simulink model "pil_testing"  (R2016a)
settings: Solver=FixedStepAuto  StartTime=0.0  StopTime=inf  FixedStep=0.05  RelTol=1e-3
undefined symbols (not defined in the file): Serial_Port, Standard_Devices
libraries: sldrtlib x2
settings Model: SimulationMode=external  Creator=aless  LastModifiedBy=aless
settings SolverCC: EnableConcurrentExecution=on
settings DataIOCC: SaveFormat=StructureWithTime  SignalLogging=off  DSMLogging=off
settings OptimizationCC: BlockReduction=off  DefaultUnderspecifiedDataType=single  OptimizeBlockIOStorage=off  BufferReuse=off  GlobalBufferReuse=off  ExpressionFolding=off  LocalBlockOutputs=off
settings DebuggingCC: MultiTaskRateTransMsg=warning
settings HardwareCC: ProdBitPerLong=64  ProdLargestAtomicFloat=None  ProdHWDeviceType=Intel->x86-64  TargetBitPerLong=64  TargetBitPerPointer=64  TargetIntDivRoundTo=Zero  TargetEndianess=LittleEndian  TargetWordSize=64  TargetHWDeviceType=Intel->x86-64
settings RTWCC: SystemTargetFile=sldrt.tlc  TemplateMakefile=sldrt.tmf  Description=Simulink Desktop Real-Time  RTWVerbose=off  RTWCompilerOptimization=on
settings CodeAppCC: ForceParamTrailComments=on  MaxIdLength=95  OperatorAnnotations=on  MATLABSourceComments=on
settings SimulinkDesktopRealTimeCC: TargetPreCompLibLocation=C:\Program Files\MATLAB\R2016a\toolbox\sldrt\lib\win64  TargetLangStandard=C89/C90 (ANSI)  SupportVariableSizeSignals=off

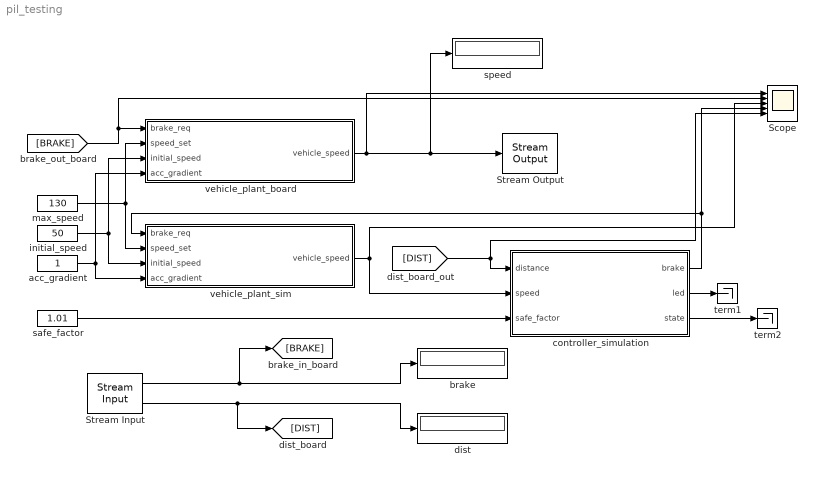
== system pil_testing ==
  Scope : Scope  NumInputPorts=5
  Stream Input : sldrtlib/Stream Input  SampleTime=0.1  MaxMissedTicks=10  ShowMissedTicks=off  YieldWhenWaiting=off  DrvName=Standard_Devices/Serial_Port  DrvAddress=5  DrvOptions=[9600 8 0 0 0 0 0 0]  DataTypes={'uint8','uint8'}  FormatString='%d %d'  Terminator='\n'  ShowReady=off  ShowError=off
      settings: AttributesFormatString=Standard Devices\nSerial Port [5h]
  Stream Output : sldrtlib/Stream Output  SampleTime=0.1  MaxMissedTicks=10  ShowMissedTicks=off  YieldWhenWaiting=off  DrvName=Standard_Devices/Serial_Port  DrvAddress=5  DrvOptions=[9600 8 0 0 0 0 0 0]  PortSizes=1  FormatString='%d\r'  ShowReady=off  ShowError=off  InitialValue=[]  FinalValue=[]
      settings: AttributesFormatString=Standard Devices\nSerial Port [5h]
  acc_gradient : Constant
  brake : Display
  controller_simulation : Subsystem
  dist : Display
  initial_speed : Constant  Value=50
  max_speed : Constant  Value=130
  safe_factor : Constant  Value=1.01
  speed : Display
  term1 : Terminator
  term2 : Terminator
  vehicle_plant_board : Subsystem
  vehicle_plant_sim : Subsystem
  wires:
  [BRAKE] -> vehicle_plant_board/1(brake_req), Scope/2
  safe_factor/1 -> controller_simulation/3(safe_factor)
  vehicle_plant_sim/1(vehicle_speed) -> controller_simulation/2(speed), Scope/3
  controller_simulation/2(led) -> term1/1
  controller_simulation/3(state) -> term2/1
  controller_simulation/1(brake) -> vehicle_plant_sim/1(brake_req), Scope/4
  vehicle_plant_board/1(vehicle_speed) -> speed/1, Stream Output/1, Scope/1
  max_speed/1 -> vehicle_plant_board/2(speed_set), vehicle_plant_sim/2(speed_set)
  initial_speed/1 -> vehicle_plant_board/3(initial_speed), vehicle_plant_sim/3(initial_speed)
  acc_gradient/1 -> vehicle_plant_board/4(acc_gradient), vehicle_plant_sim/4(acc_gradient)
  [DIST] -> controller_simulation/1(distance), Scope/5
  Stream Input/1 -> [BRAKE], brake/1
  Stream Input/2 -> dist/1, [DIST]

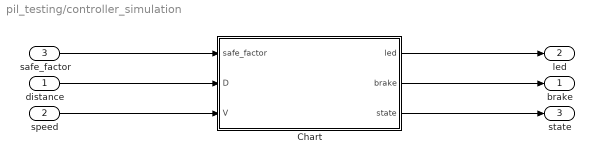
== system pil_testing/controller_simulation ==
  distance : Inport
  speed : Inport  Port=2
  safe_factor : Inport  Port=3
  Chart : Stateflow chart  TreatAsAtomicUnit=on
  brake : Outport
  led : Outport  Port=2
  state : Outport  Port=3
  wires:
  distance/1 -> Chart/2(D)
  speed/1 -> Chart/3(V)
  safe_factor/1 -> Chart/1(safe_factor)
  Chart/1(led) -> led/1
  Chart/2(brake) -> brake/1
  Chart/3(state) -> state/1

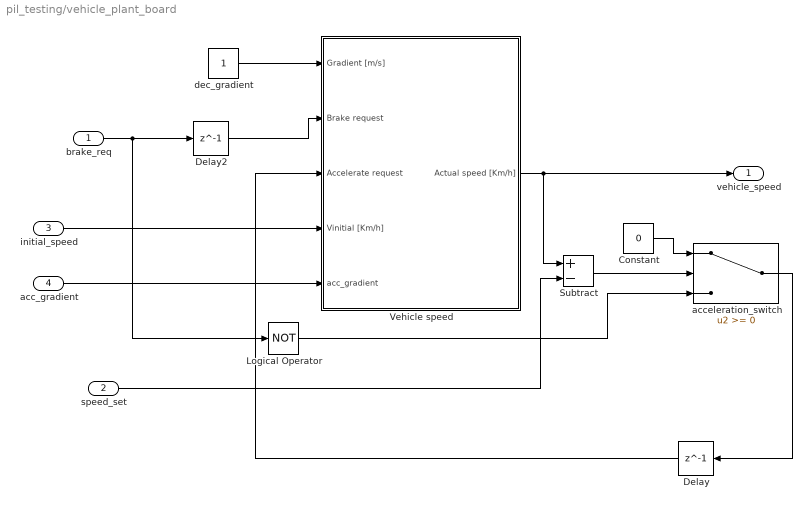
== system pil_testing/vehicle_plant_board ==
  brake_req : Inport
  speed_set : Inport  Port=2
  initial_speed : Inport  Port=3
  acc_gradient : Inport  Port=4
  Constant : Constant  Value=0
  Delay : Delay  DelayLength=1  InitialCondition=0
  Delay2 : Delay  DelayLength=1  InitialCondition=0
  Logical Operator : Logic  Operator=NOT  AllPortsSameDT=off  OutDataTypeStr=boolean
  Subtract : Sum  Inputs=+-
  Vehicle speed : Subsystem
  acceleration_switch : Switch  RndMeth=Nearest
  dec_gradient : Constant
  vehicle_speed : Outport
  wires:
  dec_gradient/1 -> Vehicle speed/1(Gradient [m/s])
  initial_speed/1 -> Vehicle speed/4(Vinitial [Km/h])
  Vehicle speed/1(Actual speed [Km/h]) -> vehicle_speed/1, Subtract/1
  Constant/1 -> acceleration_switch/1
  brake_req/1 -> Logical Operator/1, Delay2/1
  acceleration_switch/1 -> Delay/1
  Subtract/1 -> acceleration_switch/2
  speed_set/1 -> Subtract/2
  Delay2/1 -> Vehicle speed/2(Brake request)
  Logical Operator/1 -> acceleration_switch/3
  acc_gradient/1 -> Vehicle speed/5(acc_gradient)
  Delay/1 -> Vehicle speed/3(Accelerate request)

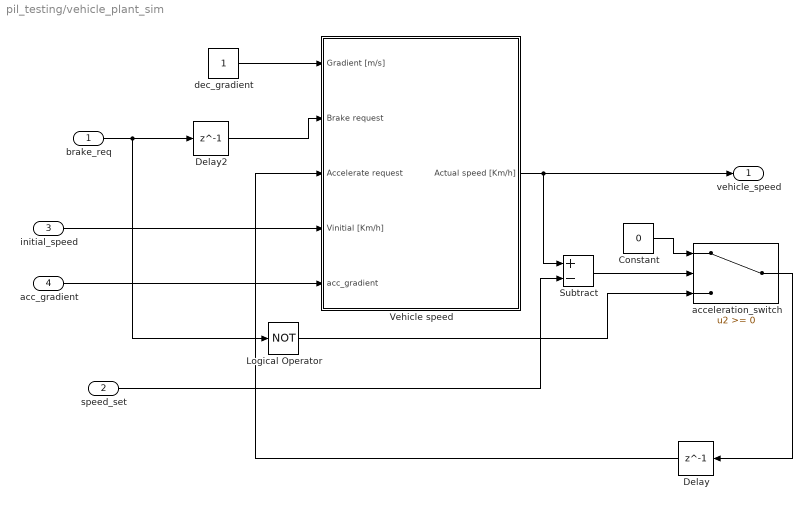
== system pil_testing/vehicle_plant_sim ==
  brake_req : Inport
  speed_set : Inport  Port=2
  initial_speed : Inport  Port=3
  acc_gradient : Inport  Port=4
  Constant : Constant  Value=0
  Delay : Delay  DelayLength=1  InitialCondition=0
  Delay2 : Delay  DelayLength=1  InitialCondition=0
  Logical Operator : Logic  Operator=NOT  AllPortsSameDT=off  OutDataTypeStr=boolean
  Subtract : Sum  Inputs=+-
  Vehicle speed : Subsystem
  acceleration_switch : Switch  RndMeth=Nearest
  dec_gradient : Constant
  vehicle_speed : Outport
  wires:
  dec_gradient/1 -> Vehicle speed/1(Gradient [m/s])
  initial_speed/1 -> Vehicle speed/4(Vinitial [Km/h])
  Vehicle speed/1(Actual speed [Km/h]) -> vehicle_speed/1, Subtract/1
  Constant/1 -> acceleration_switch/1
  brake_req/1 -> Logical Operator/1, Delay2/1
  acceleration_switch/1 -> Delay/1
  Subtract/1 -> acceleration_switch/2
  speed_set/1 -> Subtract/2
  Delay2/1 -> Vehicle speed/2(Brake request)
  Logical Operator/1 -> acceleration_switch/3
  acc_gradient/1 -> Vehicle speed/5(acc_gradient)
  Delay/1 -> Vehicle speed/3(Accelerate request)

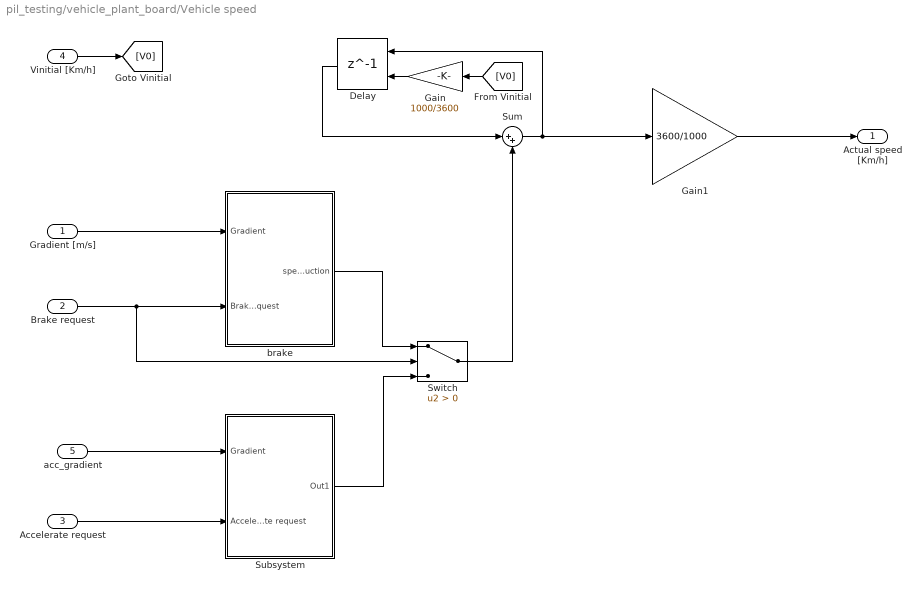
== system pil_testing/vehicle_plant_board/Vehicle speed ==
  Gradient [m/s] : Inport
  Brake request : Inport  Port=2
  Accelerate request : Inport  Port=3
  Vinitial [Km/h] : Inport  Port=4
  acc_gradient : Inport  Port=5
  Delay : Delay  DelayLength=1  InitialConditionSource=Input port  InitialCondition=0
      settings: InputPortMap=u0,p4
  Gain : Gain  Gain=1000/3600
  Gain1 : Gain  Gain=3600/1000
  Subsystem : Subsystem
  Sum : Sum  Inputs=|++
  Switch : Switch  Criteria=u2 > Threshold
  brake : Subsystem
  Actual speed [Km/h] : Outport
  wires:
  Brake request/1 -> Switch/2, brake/2(Brake request)
  Gradient [m/s]/1 -> brake/1(Gradient)
  Gain/1 -> Delay/2
  Subsystem/1(Out1) -> Switch/3
  Gain1/1 -> Actual speed [Km/h]/1
  Switch/1 -> Sum/2
  Accelerate request/1 -> Subsystem/2(Acceleate request)
  brake/1(speed_reduction) -> Switch/1
  Sum/1 -> Gain1/1, Delay/1
  [V0] -> Gain/1
  Delay/1 -> Sum/1
  Vinitial [Km/h]/1 -> [V0]
  acc_gradient/1 -> Subsystem/1(Gradient)

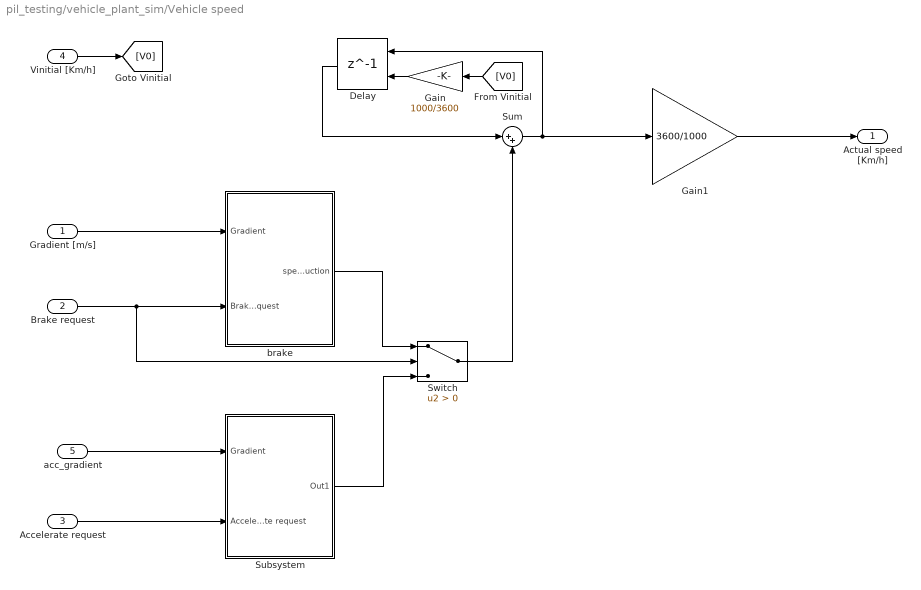
== system pil_testing/vehicle_plant_sim/Vehicle speed ==
  Gradient [m/s] : Inport
  Brake request : Inport  Port=2
  Accelerate request : Inport  Port=3
  Vinitial [Km/h] : Inport  Port=4
  acc_gradient : Inport  Port=5
  Delay : Delay  DelayLength=1  InitialConditionSource=Input port  InitialCondition=0
      settings: InputPortMap=u0,p4
  Gain : Gain  Gain=1000/3600
  Gain1 : Gain  Gain=3600/1000
  Subsystem : Subsystem
  Sum : Sum  Inputs=|++
  Switch : Switch  Criteria=u2 > Threshold
  brake : Subsystem
  Actual speed [Km/h] : Outport
  wires:
  Brake request/1 -> Switch/2, brake/2(Brake request)
  Gradient [m/s]/1 -> brake/1(Gradient)
  Gain/1 -> Delay/2
  Subsystem/1(Out1) -> Switch/3
  Gain1/1 -> Actual speed [Km/h]/1
  Switch/1 -> Sum/2
  Accelerate request/1 -> Subsystem/2(Acceleate request)
  brake/1(speed_reduction) -> Switch/1
  Sum/1 -> Gain1/1, Delay/1
  [V0] -> Gain/1
  Delay/1 -> Sum/1
  Vinitial [Km/h]/1 -> [V0]
  acc_gradient/1 -> Subsystem/1(Gradient)

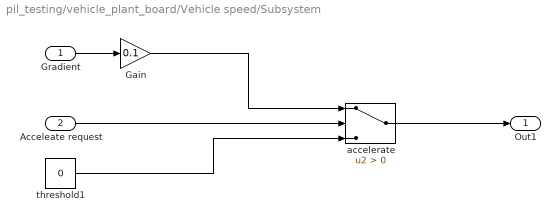
== system pil_testing/vehicle_plant_board/Vehicle speed/Subsystem ==
  Gradient : Inport
  Acceleate request : Inport  Port=2
  Gain : Gain  Gain=0.1
  accelerate : Switch  Criteria=u2 > Threshold
  threshold1 : Constant  Value=0
  Out1 : Outport
  wires:
  accelerate/1 -> Out1/1
  Acceleate request/1 -> accelerate/2
  Gradient/1 -> Gain/1
  threshold1/1 -> accelerate/3
  Gain/1 -> accelerate/1

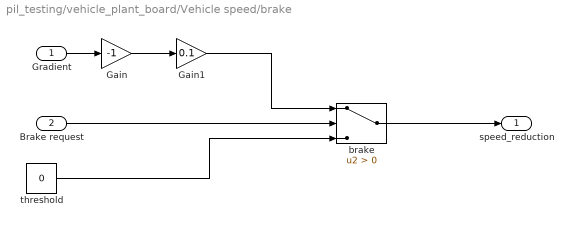
== system pil_testing/vehicle_plant_board/Vehicle speed/brake ==
  Gradient : Inport
  Brake request : Inport  Port=2
  Gain : Gain  Gain=-1
  Gain1 : Gain  Gain=0.1
  brake : Switch  Criteria=u2 > Threshold
  threshold : Constant  Value=0
  speed_reduction : Outport
  wires:
  Gain/1 -> Gain1/1
  Gradient/1 -> Gain/1
  Gain1/1 -> brake/1
  Brake request/1 -> brake/2
  threshold/1 -> brake/3
  brake/1 -> speed_reduction/1

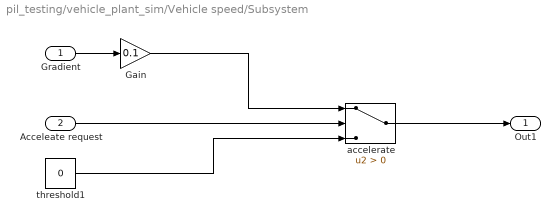
== system pil_testing/vehicle_plant_sim/Vehicle speed/Subsystem ==
  Gradient : Inport
  Acceleate request : Inport  Port=2
  Gain : Gain  Gain=0.1
  accelerate : Switch  Criteria=u2 > Threshold
  threshold1 : Constant  Value=0
  Out1 : Outport
  wires:
  accelerate/1 -> Out1/1
  Acceleate request/1 -> accelerate/2
  Gradient/1 -> Gain/1
  threshold1/1 -> accelerate/3
  Gain/1 -> accelerate/1

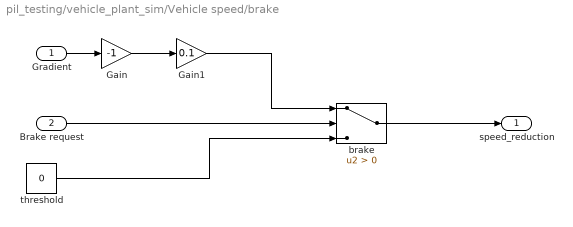
== system pil_testing/vehicle_plant_sim/Vehicle speed/brake ==
  Gradient : Inport
  Brake request : Inport  Port=2
  Gain : Gain  Gain=-1
  Gain1 : Gain  Gain=0.1
  brake : Switch  Criteria=u2 > Threshold
  threshold : Constant  Value=0
  speed_reduction : Outport
  wires:
  Gain/1 -> Gain1/1
  Gradient/1 -> Gain/1
  Gain1/1 -> brake/1
  Brake request/1 -> brake/2
  threshold/1 -> brake/3
  brake/1 -> speed_reduction/1

== stateflow chart pil_testing/controller_simulation/Chart ==
  state INIT_STATE
    en: brake = uint8(0),
    led = uint8(0),
    state = uint8(0);
  state UNSAFE_DISTANCE
    en: brake = uint8(1);
    state LED_ON
      en: led = uint8(1);
    state LED_OFF
      en: led = uint8(0);
    (default) -> LED_ON
    LED_OFF -> LED_ON : after(1/(1+V^2/100-D), msec)
    LED_ON -> LED_OFF : after(1/(1+V^2/100-D), msec)
  state SAFE_DISTANCE
    en: brake = uint8(0),
    led = uint8(0);
  (default) -> INIT_STATE
  INIT_STATE -> UNSAFE_DISTANCE [order 2] : [D <= (V^2)/100]
  INIT_STATE -> SAFE_DISTANCE [order 1] : [D > (V^2)/100]
  SAFE_DISTANCE -> UNSAFE_DISTANCE : [D <= (V^2)/100]
  UNSAFE_DISTANCE -> SAFE_DISTANCE : [D > (V^2)/100 * safe_factor]
  data: led output; safe_factor input; brake output; D input; V input; state output
